simulink model "sf_tlat"  (R2017b)
settings: Solver=ode45  StartTime=0.0  StopTime=100  RelTol=1e-3  EnableMultiTasking=on
settings Model: FPTRunName=Active  ExtModeAutoUpdateStatusClock=off  Creator=The MathWorks, Inc.  LastModifiedBy=The MathWorks, Inc.
settings DataIOCC: LimitDataPoints=on  SaveFormat=Array
settings OptimizationCC: BooleanDataType=off  ExpressionDepthLimit=2147483647  InitFltsAndDblsToZero=on  EfficientMapNaN2IntZero=off  LifeSpan=inf
settings DebuggingCC: SaveWithParameterizedLinksMsg=none  UnderspecifiedInitializationDetection=Classic  MergeDetectMultiDrivingBlocksExec=none  SignalResolutionControl=TryResolveAllWithWarning  MultiTaskDSMMsg=warning  MultiTaskCondExecSysMsg=none  FcnCallInpInsideContextMsg=warning  StateNameClashWarn=warning  StrictBusMsg=None  SFUnexpectedBacktrackingDiag=warning  SFNoUnconditionalDefaultTransitionDiag=warning  SFExecutionAtInitializationDiag=none
settings HardwareCC: ProdBitPerPointer=32  ProdBitPerSizeT=32  ProdBitPerPtrDiffT=32  ProdLargestAtomicFloat=None  ProdIntDivRoundTo=Undefined  ProdEndianess=Unspecified  ProdWordSize=32  ProdHWDeviceType=32-bit Generic  TargetUnknown=on
settings ModelReferenceCC: PropagateSignalLabelsOutOfModel=off
settings SFSimCC: SimParseCustomCode=off
settings CodeAppCC: StateflowObjectComments=on
settings GRTTargetCC: TargetFcnLib=ansi_tfl_tmw.mat  TargetLangStandard=C89/C90 (ANSI)  GeneratePreprocessorConditionals=Disable all  CombineOutputUpdateFcns=off  GRTInterface=on
settings ConfigComp: CovMetricSettings=dcmtr  CovHtmlReporting=on  CovSaveCumulativeToWorkspaceVar=on  CovSaveSingleToWorkspaceVar=on  CovExternalEMLEnable=off  CovSFcnEnable=off

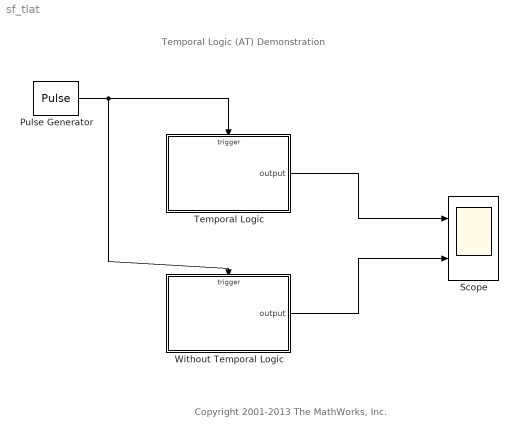
== system sf_tlat ==
  note: Temporal Logic (AT) Demonstration
  note: Copyright 2001-2013 The MathWorks, Inc.
  Pulse Generator : DiscretePulseGenerator  PulseType=Time based  Period=1  PulseWidth=50
  Scope : Scope  NumInputPorts=2
  Temporal Logic : Stateflow chart  TreatAsAtomicUnit=on
  Without Temporal Logic : Stateflow chart  TreatAsAtomicUnit=on
  wires:
  Pulse Generator/1 -> Temporal Logic/Trigger, Without Temporal Logic/Trigger
  Temporal Logic/1(output) -> Scope/1
  Without Temporal Logic/1(output) -> Scope/2

== stateflow chart sf_tlat/Temporal Logic ==
  state State
    a=5;
    on at(a,event):output=1;
    on at(2*a,event):output=0;
  (default) -> State
  State -> (junction 5) : at(6*a,event)
  (junction 5) -> State : {output=-1;}
  data: output output double; a local double
  events: event input RISING_EDGE_EVENT

== stateflow chart sf_tlat/Without Temporal Logic ==
  state A
    en: count = 1;
    A -> A [order 1] : {count++;a=count;}
  state B
    en:count=a+1;
    B -> B [order 1] : {count++;}
  state C
    en:count=2*a+1;
    C -> C [order 1] : {count++;}
  (default) -> A
  A -> B [order 1] : [count==5]{output=1;}
  C -> A [order 1] : [count==6*a]{output=-1;}
  B -> C [order 1] : [count==2*a]{output=0;}
  data: count local double; output output double; a local double
  events: control input RISING_EDGE_EVENT
